simulink model "lqr_control_model"  (R2022b)
settings: Solver=VariableStepAuto  StartTime=0.0  StopTime=20  RelTol=1e-3
undefined symbols (not defined in the file): Lqr, Reqr, RunArg, SS, Stm
settings Model: Creator=guila  LastModifiedBy=guila

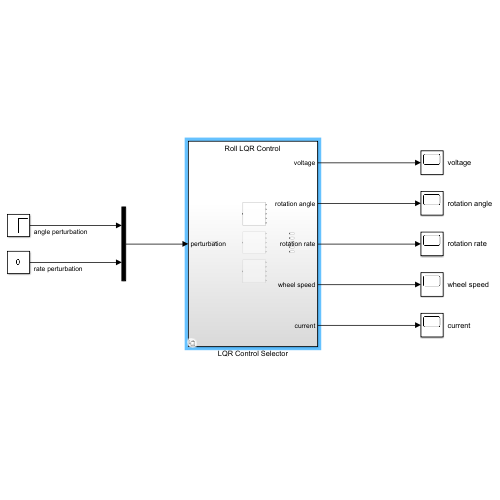
[thumbnail: Simulink's stored preview of the top-level diagram]
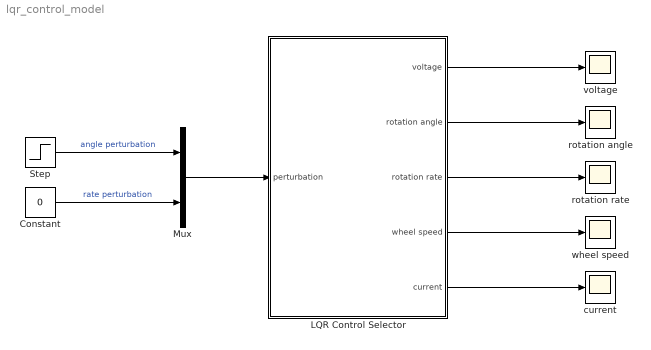
== system lqr_control_model ==
  Constant : Constant  Value=0
  LQR Control Selector : Subsystem  Variant=on
  Mux : Mux  Inputs=2
  Step : Step  SampleTime=0
  current : Scope
  rotation angle : Scope
  rotation rate : Scope
  voltage : Scope
  wheel speed : Scope
  wires:
  LQR Control Selector/1(voltage) -> voltage/1
  LQR Control Selector/2(rotation angle) -> rotation angle/1
  LQR Control Selector/3(rotation rate) -> rotation rate/1
  LQR Control Selector/4(wheel speed) -> wheel speed/1
  LQR Control Selector/5(current) -> current/1
  Step/1 -> Mux/1  "angle perturbation"
  Constant/1 -> Mux/2  "rate perturbation"
  Mux/1 -> LQR Control Selector/1(perturbation)

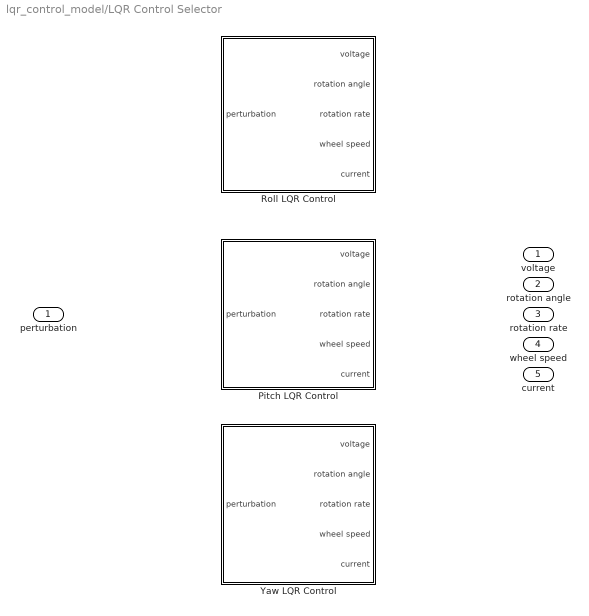
== system lqr_control_model/LQR Control Selector ==
  perturbation : Inport
  Pitch LQR Control : Subsystem  VariantControl=strcmp(RunArg.selsim, 'pitch')
  Roll LQR Control : Subsystem  VariantControl=strcmp(RunArg.selsim, 'roll')
  Yaw LQR Control : Subsystem  VariantControl=strcmp(RunArg.selsim, 'yaw')
  voltage : Outport
  rotation angle : Outport  Port=2
  rotation rate : Outport  Port=3
  wheel speed : Outport  Port=4
  current : Outport  Port=5

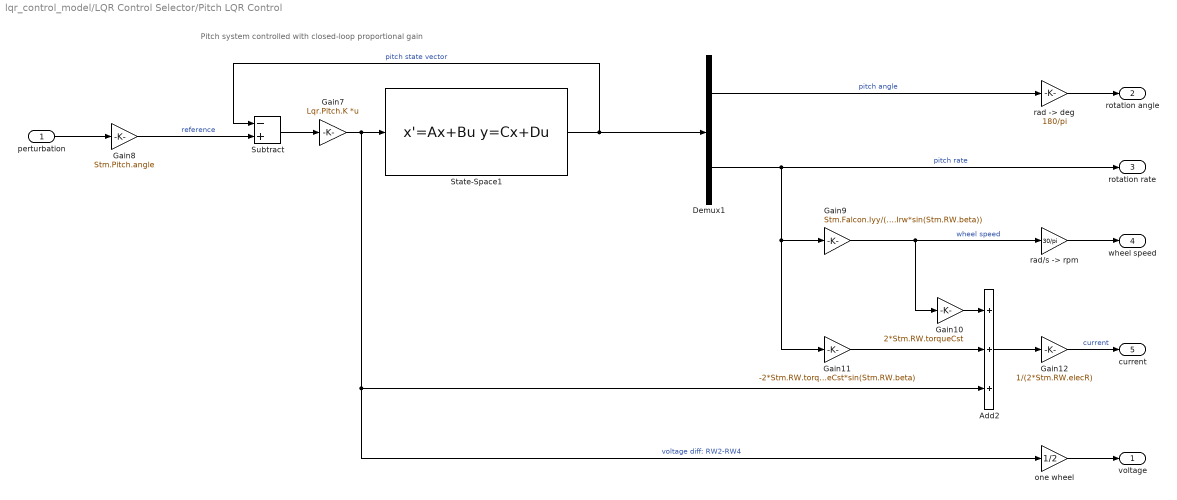
== system lqr_control_model/LQR Control Selector/Pitch LQR Control ==
  note: Pitch system controlled with closed-loop proportional gain
  perturbation : Inport
  Add2 : Sum  Inputs=+++
  Demux1 : Demux  Outputs=2
  Gain10 : Gain  Gain=2*Stm.RW.torqueCst
  Gain11 : Gain  Gain=-2*Stm.RW.torqueCst*sin(Stm.RW.beta)
  Gain12 : Gain  Gain=1/(2*Stm.RW.elecR)
  Gain7 : Gain  Gain=Lqr.Pitch.K  Multiplication=Matrix(K*u) (u vector)
  Gain8 : Gain  Gain=Stm.Pitch.angle
  Gain9 : Gain  Gain=Stm.Falcon.Iyy/(2*Reqr.Sizing.Irw*sin(Stm.RW.beta))
  State-Space1 : StateSpace  A=SS.Pitch.A  B=SS.Pitch.B  C=SS.Pitch.C  D=SS.Pitch.D  InitialCondition=0
  Subtract : Sum  Inputs=-+
  one wheel : Gain  Gain=1/2
  "rad -> deg" : Gain  Gain=180/pi
  "rad/s -> rpm" : Gain  Gain=30/pi
  voltage : Outport
  rotation angle : Outport  Port=2
  rotation rate : Outport  Port=3
  wheel speed : Outport  Port=4
  current : Outport  Port=5
  wires:
  Gain8/1 -> Subtract/2  "reference"
  Gain9/1 -> Gain10/1, "rad/s -> rpm"/1  "wheel speed"
  Demux1/2 -> rotation rate/1, Gain11/1, Gain9/1  "pitch rate"
  Demux1/1 -> "rad -> deg"/1  "pitch angle"
  "rad -> deg"/1 -> rotation angle/1
  one wheel/1 -> voltage/1
  Add2/1 -> Gain12/1
  Subtract/1 -> Gain7/1
  perturbation/1 -> Gain8/1
  "rad/s -> rpm"/1 -> wheel speed/1
  Gain12/1 -> current/1  "current"
  Gain11/1 -> Add2/2
  Gain10/1 -> Add2/1
  State-Space1/1 -> Subtract/1, Demux1/1  "pitch state vector"
  Gain7/1 -> State-Space1/1, one wheel/1, Add2/3  "voltage diff: RW2-RW4"

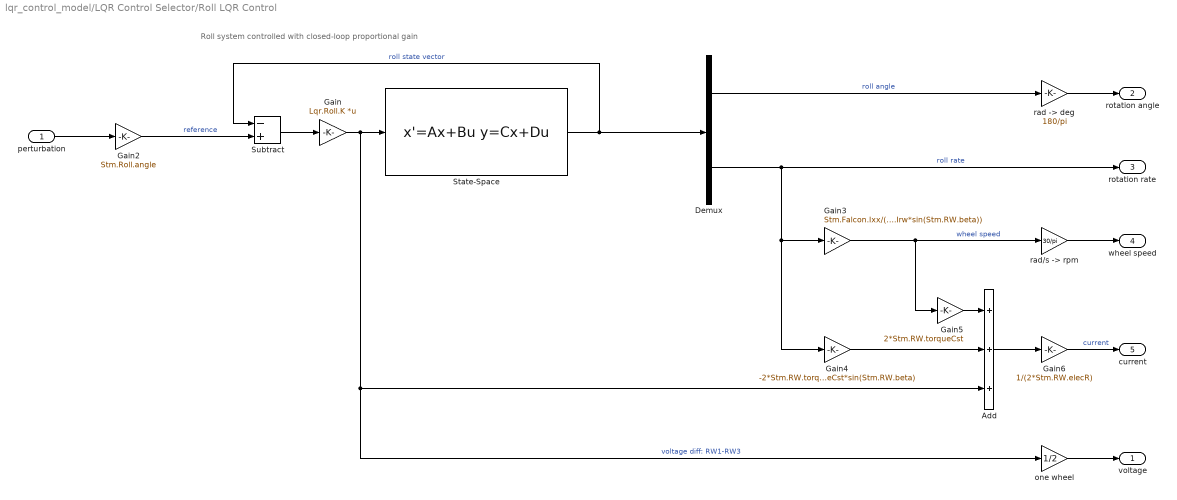
== system lqr_control_model/LQR Control Selector/Roll LQR Control ==
  note: Roll system controlled with closed-loop proportional gain
  perturbation : Inport
  Add : Sum  Inputs=+++
  Demux : Demux  Outputs=2
  Gain : Gain  Gain=Lqr.Roll.K  Multiplication=Matrix(K*u) (u vector)
  Gain2 : Gain  Gain=Stm.Roll.angle
  Gain3 : Gain  Gain=Stm.Falcon.Ixx/(2*Reqr.Sizing.Irw*sin(Stm.RW.beta))
  Gain4 : Gain  Gain=-2*Stm.RW.torqueCst*sin(Stm.RW.beta)
  Gain5 : Gain  Gain=2*Stm.RW.torqueCst
  Gain6 : Gain  Gain=1/(2*Stm.RW.elecR)
  State-Space : StateSpace  A=SS.Roll.A  B=SS.Roll.B  C=SS.Roll.C  D=SS.Roll.D  InitialCondition=0
  Subtract : Sum  Inputs=-+
  one wheel : Gain  Gain=1/2
  "rad -> deg" : Gain  Gain=180/pi
  "rad/s -> rpm" : Gain  Gain=30/pi
  voltage : Outport
  rotation angle : Outport  Port=2
  rotation rate : Outport  Port=3
  wheel speed : Outport  Port=4
  current : Outport  Port=5
  wires:
  Gain4/1 -> Add/2
  Gain5/1 -> Add/1
  State-Space/1 -> Subtract/1, Demux/1  "roll state vector"
  Demux/1 -> "rad -> deg"/1  "roll angle"
  Demux/2 -> rotation rate/1, Gain4/1, Gain3/1  "roll rate"
  perturbation/1 -> Gain2/1
  Gain3/1 -> Gain5/1, "rad/s -> rpm"/1  "wheel speed"
  "rad -> deg"/1 -> rotation angle/1
  Add/1 -> Gain6/1
  "rad/s -> rpm"/1 -> wheel speed/1
  Gain6/1 -> current/1  "current"
  one wheel/1 -> voltage/1
  Gain/1 -> State-Space/1, one wheel/1, Add/3  "voltage diff: RW1-RW3"
  Subtract/1 -> Gain/1
  Gain2/1 -> Subtract/2  "reference"

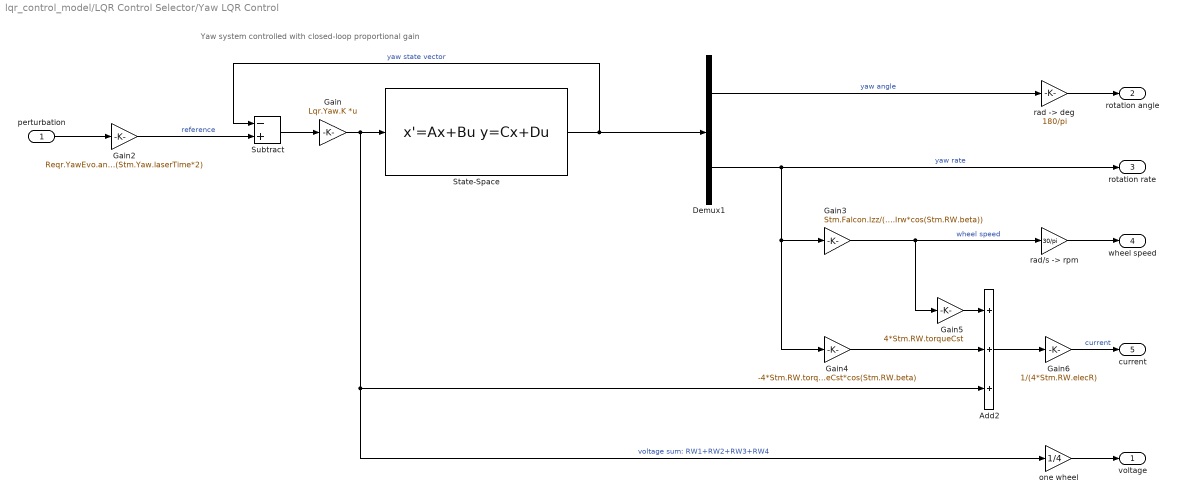
== system lqr_control_model/LQR Control Selector/Yaw LQR Control ==
  note: Yaw system controlled with closed-loop proportional gain
  perturbation : Inport
  Add2 : Sum  Inputs=+++
  Demux1 : Demux  Outputs=2
  Gain : Gain  Gain=Lqr.Yaw.K  Multiplication=Matrix(K*u) (u vector)
  Gain2 : Gain  Gain=Reqr.YawEvo.angle(Stm.Yaw.laserTime*2)
  Gain3 : Gain  Gain=Stm.Falcon.Izz/(4*Reqr.Sizing.Irw*cos(Stm.RW.beta))
  Gain4 : Gain  Gain=-4*Stm.RW.torqueCst*cos(Stm.RW.beta)
  Gain5 : Gain  Gain=4*Stm.RW.torqueCst
  Gain6 : Gain  Gain=1/(4*Stm.RW.elecR)
  State-Space : StateSpace  A=SS.Yaw.A  B=SS.Yaw.B  C=SS.Yaw.C  D=SS.Yaw.D  InitialCondition=0
  Subtract : Sum  Inputs=-+
  one wheel : Gain  Gain=1/4
  "rad -> deg" : Gain  Gain=180/pi
  "rad/s -> rpm" : Gain  Gain=30/pi
  voltage : Outport
  rotation angle : Outport  Port=2
  rotation rate : Outport  Port=3
  wheel speed : Outport  Port=4
  current : Outport  Port=5
  wires:
  "rad/s -> rpm"/1 -> wheel speed/1
  "rad -> deg"/1 -> rotation angle/1
  Gain4/1 -> Add2/2
  Gain5/1 -> Add2/1
  Gain/1 -> State-Space/1, one wheel/1, Add2/3  "voltage sum: RW1+RW2+RW3+RW4"
  Demux1/2 -> rotation rate/1, Gain4/1, Gain3/1  "yaw rate"
  Gain6/1 -> current/1  "current"
  perturbation/1 -> Gain2/1
  Gain3/1 -> Gain5/1, "rad/s -> rpm"/1  "wheel speed"
  Gain2/1 -> Subtract/2  "reference"
  Add2/1 -> Gain6/1
  one wheel/1 -> voltage/1
  Subtract/1 -> Gain/1
  State-Space/1 -> Subtract/1, Demux1/1  "yaw state vector"
  Demux1/1 -> "rad -> deg"/1  "yaw angle"
